simulink model "tutorial17_leadlag"  (R2025a)
settings: Solver=VariableStepAuto  StartTime=0.0  StopTime=10.0  RelTol=1e-3
settings Model: Creator=xing2  LastModifiedBy=xing2

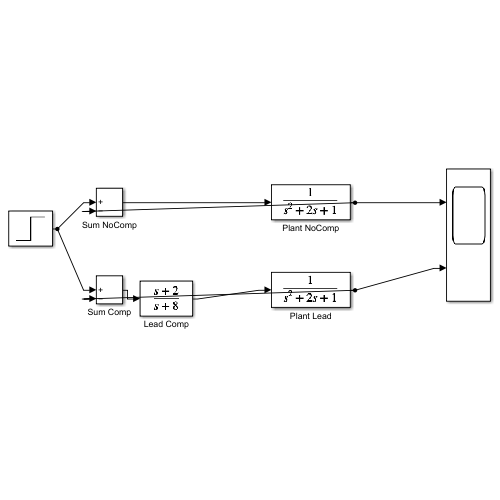
[thumbnail: Simulink's stored preview of the top-level diagram]
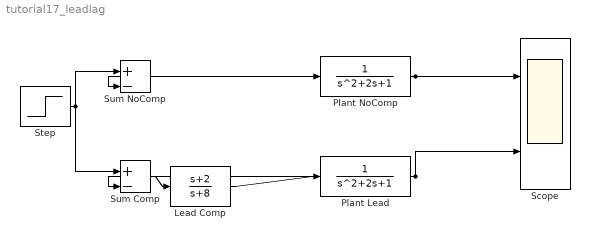
== system tutorial17_leadlag ==
  Lead Comp : TransferFcn  Numerator=[1 2]  Denominator=[1 8]
  Plant Lead : TransferFcn
  Plant NoComp : TransferFcn
  Scope : Scope  NumInputPorts=2
  Step : Step  Time=0.5  SampleTime=0
  Sum Comp : Sum  Inputs=|+-
  Sum NoComp : Sum  Inputs=|+-
  wires:
  Step/1 -> Sum NoComp/1, Sum Comp/1
  Sum NoComp/1 -> Plant NoComp/1
  Plant NoComp/1 -> Scope/1, Sum NoComp/2
  Sum Comp/1 -> Lead Comp/1
  Lead Comp/1 -> Plant Lead/1
  Plant Lead/1 -> Scope/2, Sum Comp/2
